simulink model "TrayectoriaPurePursuitS"  (R2023b)
settings: Solver=FixedStepAuto  StartTime=0.0  StopTime=20  RelTol=1e-3  EnableMultiTasking=on
model workspace (MAT data in the model file):
  d = 0.175
libraries: robotalgslib x1
settings Model: ExtModeTrigDuration=2  Creator=Enrique  LastModifiedBy=Enrique
settings OptimizationCC: EnhancedBackFolding=on  PassReuseOutputArgsAs=Individual arguments  ZeroExternalMemoryAtStartup=off  ZeroInternalMemoryAtStartup=off  MaxStackSize=64  OptimizeBlockOrder=speed  DifferentSizesBufferReuse=on  EfficientTunableParamExpr=on
settings DebuggingCC: AlgebraicLoopMsg=none  ParameterTunabilityLossMsg=error
settings HardwareCC: ProdBitPerInt=16  ProdBitPerPointer=16  ProdBitPerSizeT=16  ProdBitPerPtrDiffT=16  ProdLargestAtomicFloat=None  ProdWordSize=8  ProdHWDeviceType=Atmel->AVR  UseEmbeddedCoderFeatures=off  UseSimulinkCoderFeatures=off
settings SFSimCC: MATLABDynamicMemAlloc=off
settings RTWCC: Description=Embedded Coder  SystemTargetFile=ert.tlc  HardwareBoard=Arduino Mega 2560  TemplateMakefile=ert_default_tmf  Toolchain=Arduino AVR  BuildConfiguration=Faster Runs
settings CodeAppCC: ForceParamTrailComments=on  IgnoreCustomStorageClasses=off  OperatorAnnotations=on  SimulinkDataObjDesc=on  SFDataObjDesc=on  InsertBlockDesc=on
settings ERTTargetCC: SupportContinuousTime=on  SupportNonInlinedSFcns=on  SupportVariableSizeSignals=on  ExtModeTransport=3  ExtModeStaticAlloc=on  ExtModeAutomaticAllocSize=off  ExtModeStaticAllocSize=2048  ExtModeMexFile=ext_xcp  ExtModeIntrfLevel=Level2 - Open

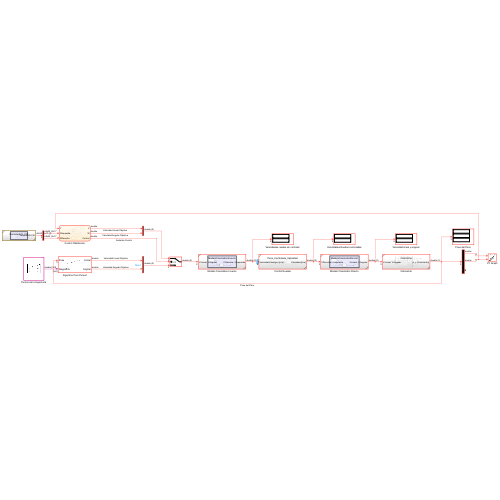
[thumbnail: Simulink's stored preview of the top-level diagram]
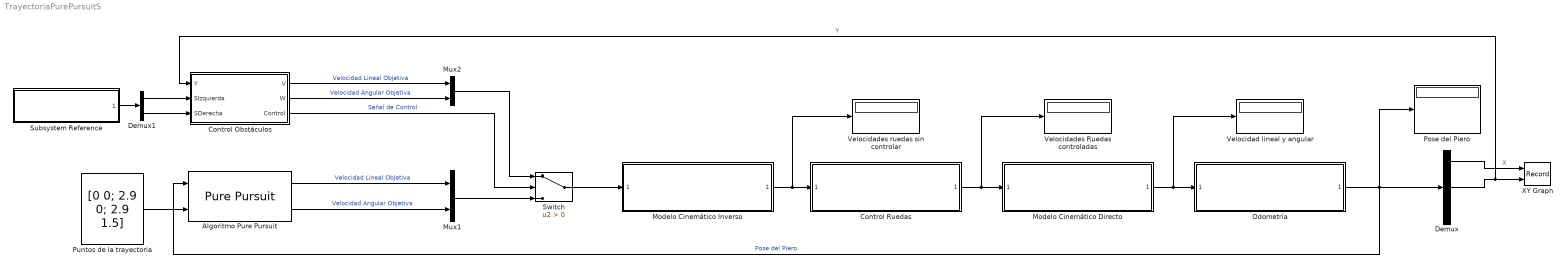
== system TrayectoriaPurePursuitS ==
  Algoritmo Pure Pursuit : robotalgslib/Pure Pursuit  DesiredLinearVelocity=0.22  MaxAngularVelocity=0.75  LookaheadDistance=0.35  TargetDirPort=off  SimulateUsing=Code generation
      settings: LibrarySourceBlock=robotmobilelib/Pure Pursuit
  Control Obstáculos : Stateflow chart  TreatAsAtomicUnit=on
  Control Ruedas : Subsystem  ReferencedSubsystem=Piero_Controlado_Velocidad
  Demux : Demux  Outputs=3
  Demux1 : Demux  Outputs=2
  Modelo Cinemático Directo : Subsystem  ReferencedSubsystem=ModeloCinematicoDirecto
  Modelo Cinemático Inverso : Subsystem  ReferencedSubsystem=ModeloCinematicoInverso
  Mux1 : Mux  Inputs=2
  Mux2 : Mux  Inputs=2
  Odometría : Subsystem  ReferencedSubsystem=Odometria
  Pose del Piero : Display
  Puntos de la trayectoria : Constant  Value=[0 0; 2.9 0; 2.9 1.5]
  Subsystem Reference : Subsystem  ReferencedSubsystem=SensoresUS_016
  Switch : Switch  Criteria=u2 > Threshold  SaturateOnIntegerOverflow=off  InputSameDT=off
  Velocidad lineal y angular : Display
  Velocidades Ruedas controladas : Display
  Velocidades ruedas sin controlar : Display
  XY Graph : Record  FileSettingsInternal="{\"entries\":[{\"content\":{\"excelSettings\":{\"content\":{},\"type\":\"Streamout.ExcelSettings\"}},\"type\":\"Streamout.FileSettingStorage\",\"uuid\":\"\"}],\"packageUris\":[\"http:\\/\\/schema.mathworks.com\\/mf0\\/streamout_blocks\\/R2020a\"],\"version\":\"1.0\"}"  Layout=[1 1]  SignalsInternal="{\"entries\":[{\"content\":{\"signals\":[{\"content\":{\"blockPath\":[],\"dimensions\":[1],\"domain\":\"\",\"lineColor\":\"#a2142f\",\"plots\":[ 1 ],\"port\":1,\"sid\":[\"26\"],\"signalID\":1,\"signalName\":\"X\"},\"type\":\"RecordBlkView.Signal\",\"uuid\":\"\"},{\"content\":{\"blockPath\":[],\"dimensions\":[1],\"domain\":\"\",\"lineColor\":\"#139fff\",\"plots\":[ 1 ],\"port\":2,\"sid\":[\"26\"],\"signalID\":2,\"signalName\":\"Y\"},\"type\":\"RecordBlkView.Signal\",\"uuid\":\"\"}]},\"type\":\"RecordBlkView.InputSignals\",\"uuid\":\"\"}],\"packageUris\":[\"http:\\/\\/schema.mathworks.com\\/mf0\\/streamout_blocks\\/R2020a\"],\"version\":\"1.0\"}"  VisualizationBindings="{\"xyplotplugin\":{\"info\":[{\"series\":[{\"bindingParametersList\":[{\"parameter\":\"X-Axis\",\"signalID\":1,\"signalName\":\"X\"},{\"parameter\":\"Y-Axis\",\"signalID\":2,\"signalName\":\"Y\"}],\"seriesID\":0}],\"subplotID\":1}]}}"  CompatibilityTag=XY
  wires:
  Modelo Cinemático Inverso/1 -> Velocidades ruedas sin controlar/1, Control Ruedas/1
  Control Ruedas/1 -> Velocidades Ruedas controladas/1, Modelo Cinemático Directo/1
  Modelo Cinemático Directo/1 -> Velocidad lineal y angular/1, Odometría/1
  Odometría/1 -> Pose del Piero/1, Algoritmo Pure Pursuit/1, Demux/1  "Pose del Piero"
  Demux/1 -> XY Graph/1  "X"
  Algoritmo Pure Pursuit/1 -> Mux1/1  "Velocidad Lineal Objetiva"
  Demux/2 -> Control Obstáculos/1(Y), XY Graph/2  "Y"
  Puntos de la trayectoria/1 -> Algoritmo Pure Pursuit/2
  Algoritmo Pure Pursuit/2 -> Mux1/2  "Velocidad Angular Objetiva"
  Control Obstáculos/1(V) -> Mux2/1  "Velocidad Lineal Objetiva"
  Control Obstáculos/2(W) -> Mux2/2  "Velocidad Angular Objetiva"
  Switch/1 -> Modelo Cinemático Inverso/1
  Mux1/1 -> Switch/3
  Control Obstáculos/3(Control) -> Switch/2  "Señal de Control"
  Mux2/1 -> Switch/1
  Subsystem Reference/1 -> Demux1/1
  Demux1/1 -> Control Obstáculos/2(SIzquierda)
  Demux1/2 -> Control Obstáculos/3(SDerecha)

== stateflow chart TrayectoriaPurePursuitS/Control Obstáculos ==
  state FinTrayectoria
    V=0;
    W = 0;
    Control = 1;
  state SinObstaculos
    V = 0;
    W = 0;
    Control = 0;
  state ObstaculoIzquierda
    V = 0.1;
    W = -pi/4;
    Control = 1;
  state ObstaculoDerecha
    V = 0.1;
    W = pi/4;
    Control = 1;
  state ObstaculoFrente
    V = 0;
    W = pi/2;
    Control = 1;
  SinObstaculos -> FinTrayectoria [order 3] : [Y > 1]
  (default) -> SinObstaculos
  SinObstaculos -> ObstaculoIzquierda [order 1] : [SIzquierda < 30]
  SinObstaculos -> ObstaculoDerecha [order 2] : [SDerecha < 30]
  ObstaculoIzquierda -> SinObstaculos [order 1] : [after(1,sec)]
  ObstaculoFrente -> SinObstaculos : [after(1.5,sec)]
  ObstaculoDerecha -> SinObstaculos [order 1] : [after(1,sec)]
  ObstaculoIzquierda -> ObstaculoFrente [order 2] : [SDerecha < 15]
  ObstaculoDerecha -> ObstaculoFrente [order 2] : [SIzquierda < 15]
  data: Y input; V output; W output; Control output; SIzquierda input; SDerecha input
